simulink model "myGuyton_corrected_new"  (Simulink 6.6)
settings: Solver=ode15s  StartTime=0  StopTime=60*24*14  FixedStep=0.025  MaxStep=1  MinStep=0.00000001  RelTol=1e-1
values from neighbouring files (symbols this model uses):
  A1K = 0.5    [G92_var_decl_exp.m]
  A2K = 60    [G92_var_decl_exp.m]
  A3K = 40000    [G92_var_decl_exp.m]
  A4K = 0.1    [G92_var_decl_exp.m]
  A4K2 = 40000    [G92_var_decl_exp.m]
  AARK = 1    [G92_var_decl_exp.m]
  AARLL = 4    [G92_var_decl_exp.m]
  ADHC_IC = 1.01449    [G92_var_decl_exp.m]
  ADHINF = 0    [G92_var_decl_exp.m]
  ADHKLL = 0.2    [G92_var_decl_exp.m]
  ADHKUL = 5    [G92_var_decl_exp.m]
  ADHPAM = 0.3    [G92_var_decl_exp.m]
  ADHPUL = 85    [G92_var_decl_exp.m]
  ADHTC = 15    [G92_var_decl_exp.m]
  ADHVLL = 0.93617    [G92_var_decl_exp.m]
  ADHVUL = 2.5    [G92_var_decl_exp.m]
  AH10 = 0.333    [G92_var_decl_exp.m]
  AH11 = 1000    [G92_var_decl_exp.m]
  AH9 = 1    [G92_var_decl_exp.m]
  AHMNAR = 0.3    [G92_var_decl_exp.m]
  AHTHM = 2    [G92_var_decl_exp.m]
  AHY_IC = -0.461862    [G92_var_decl_exp.m]
  ALCLK = 0.3    [G92_var_decl_exp.m]
  ALDINF = 0    [G92_var_decl_exp.m]
  ALDKNS = 0    [G92_var_decl_exp.m]
  ALDMM = 2.5    [G92_var_decl_exp.m]
  AM1LL = 0    [G92_var_decl_exp.m]
  AM1UL = 5    [G92_var_decl_exp.m]
  AMC_IC = 1.05537    [G92_var_decl_exp.m]
  AMCSNS = 0.65    [G92_var_decl_exp.m]
  AMKM = 0.5    [G92_var_decl_exp.m]
  AMKMUL = 12    [G92_var_decl_exp.m]
  AMM1_IC = 1.00227    [G92_var_decl_exp.m]
  AMM2_IC = 1.09458    [G92_var_decl_exp.m]
  AMM4 = 0.005    [G92_var_decl_exp.m]
  AMNALL = 0.04    [G92_var_decl_exp.m]
  AMNAM = 0.8    [G92_var_decl_exp.m]
  AMNAUL = 15    [G92_var_decl_exp.m]
  AMT = 60    [G92_var_decl_exp.m]
  ANC_IC = 0.867681    [G92_var_decl_exp.m]
  ANCSNS = 0.4    [G92_var_decl_exp.m]
  ANGINF = 0    [G92_var_decl_exp.m]
  ANGKNS = 0    [G92_var_decl_exp.m]
  ANMALD = 2.5    [G92_var_decl_exp.m]
  ANMAM = 1.4    [G92_var_decl_exp.m]
  ANMARL = 0.86    [G92_var_decl_exp.m]
  ANMEM = 1.6    [G92_var_decl_exp.m]
  ANMKEL = 0.3    [G92_var_decl_exp.m]
  ANMKEM = 2    [G92_var_decl_exp.m]
  ANMLL = 0.7    [G92_var_decl_exp.m]
  ANMNAM = 1    [G92_var_decl_exp.m]
  ANMSLT = 2    [G92_var_decl_exp.m]
  ANMTM = 1.5    [G92_var_decl_exp.m]
  ANMUL = 1.8    [G92_var_decl_exp.m]
  ANPC_IC = 0.9333    [G92_var_decl_exp.m]
  ANPINF = 0    [G92_var_decl_exp.m]
  ANPKNS = 0    [G92_var_decl_exp.m]
  ANPTC = 4    [G92_var_decl_exp.m]
  ANPXAF = 1.5    [G92_var_decl_exp.m]
  ANPXUL = 10    [G92_var_decl_exp.m]
  ANT = 12    [G92_var_decl_exp.m]
  ANULL = 0.8    [G92_var_decl_exp.m]
  ANUM = 6    [G92_var_decl_exp.m]
  ANUVM = 0    [G92_var_decl_exp.m]
  ANV = 5000    [G92_var_decl_exp.m]
  ANX1_IC = 0    [G92_var_decl_exp.m]
  ANXM = 0    [G92_var_decl_exp.m]
  ANY = -0.2    [G92_var_decl_exp.m]
  AR1_IC = 1.00197    [G92_var_decl_exp.m]
  AR2_IC = 1.00306    [G92_var_decl_exp.m]
  AR3_IC = 1.05777    [G92_var_decl_exp.m]
  ARF = 0.5    [G92_var_decl_exp.m]
  ATRFBM = 0    [G92_var_decl_exp.m]
  ATRVM = 0    [G92_var_decl_exp.m]
  AU1_IC = 0.99999    [G92_var_decl_exp.m]
  AU4_IC = -0.00833091    [G92_var_decl_exp.m]
  AU6_IC = 1.00041    [G92_var_decl_exp.m]
  AUC1 = 0.3    [G92_var_decl_exp.m]
  AUDMP = 0.3    [G92_var_decl_exp.m]
  AUK = 0.004    [G92_var_decl_exp.m]
  AUL = 1.5    [G92_var_decl_exp.m]
  AULPM = 0    [G92_var_decl_exp.m]
  AUM1 = 3    [G92_var_decl_exp.m]
  AUM2 = 1    [G92_var_decl_exp.m]
  AUMAX = 5    [G92_var_decl_exp.m]
  AUMIN = 0.4    [G92_var_decl_exp.m]
  AUMK1 = 0.3    [G92_var_decl_exp.m]
  AUN1 = 0.5    [G92_var_decl_exp.m]
  AUS = 1    [G92_var_decl_exp.m]
  AUSLP = 1.5    [G92_var_decl_exp.m]
  AUTOGN = 7    [G92_var_decl_exp.m]
  AUTOK = 0.1    [G92_var_decl_exp.m]
  AUTOSN = 0.9    [G92_var_decl_exp.m]
  AUV = 0.55    [G92_var_decl_exp.m]
  AUX = 1    [G92_var_decl_exp.m]
  AUY = 0    [G92_var_decl_exp.m]
  BAROTC = 0.16    [G92_var_decl_exp.m]
  CFC = 0.01167    [G92_var_decl_exp.m]
  CKEEX = 4    [G92_var_decl_exp.m]
  CMPTSS = 2    [G92_var_decl_exp.m]
  CN2 = 0.0212    [G92_var_decl_exp.m]
  CN3_IC = 0.359907    [G92_var_decl_exp.m]
  CN7 = 0.2    [G92_var_decl_exp.m]
  CNR = 139    [G92_var_decl_exp.m]
  CPF = 0.0003    [G92_var_decl_exp.m]
  CPK = 0.000253    [G92_var_decl_exp.m]
  CPR = 40    [G92_var_decl_exp.m]
  CRRFLX = 0    [G92_var_decl_exp.m]
  CV = 0.1    [G92_var_decl_exp.m]
  DFP_IC = 1.16492e-06    [G92_var_decl_exp.m]
  DHDTR = 0.05    [G92_var_decl_exp.m]
  DIURET = 1    [G92_var_decl_exp.m]
  DR = 0    [G92_var_decl_exp.m]
  DTKA_IC = 0.0368507    [G92_var_decl_exp.m]
  DTNAR = 0.675    [G92_var_decl_exp.m]
  DTNARL = 1e-06    [G92_var_decl_exp.m]
  EARK = 1    [G92_var_decl_exp.m]
  EARLL = 24    [G92_var_decl_exp.m]
  EFAFR = 0    [G92_var_decl_exp.m]
  EXC = 1    [G92_var_decl_exp.m]
  ... (+137 more)
libraries: simulink x5
(part 1 of 3)
settings Model: Creator=Villy  LastModifiedBy=Villy
settings DataIOCC: LimitDataPoints=off  SaveOutput=off  SaveTime=off
settings DebuggingCC: SignalInfNanChecking=error  AlgebraicLoopMsg=none  ArtificialAlgebraicLoopMsg=error  SignalResolutionControl=TryResolveAll  BlockPriorityViolationMsg=error  MinStepSizeMsg=error  SolverPrmCheckMsg=error

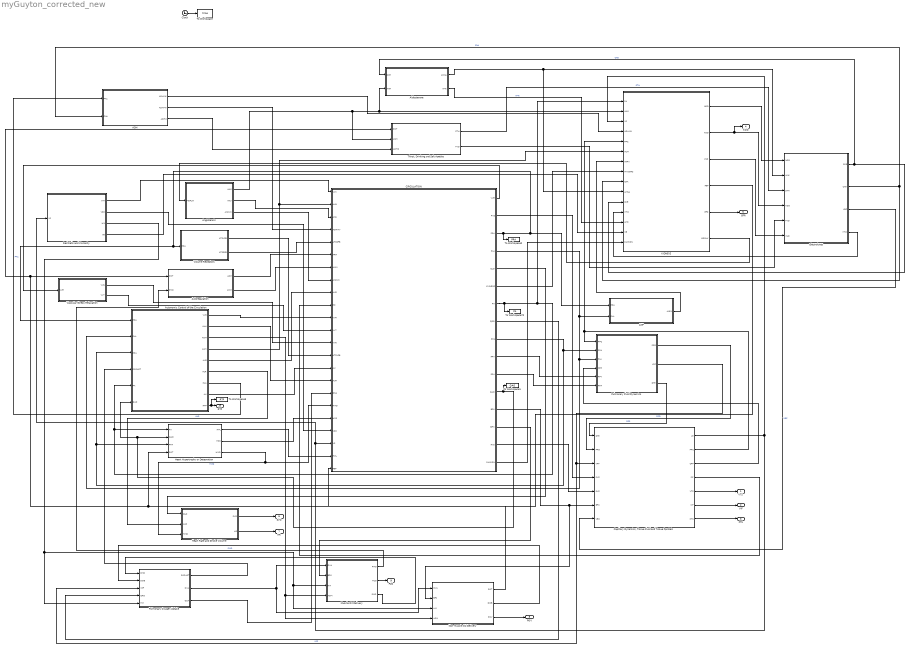
== system myGuyton_corrected_new ==
  ADH : Subsystem
      mask Display: disp('ANTIDIURETIC HORMONE')
  ANP : Subsystem
      mask Display: disp('ATRIAL NATRIURETIC PEPTIDE')
  Aldosterone : Subsystem
      mask Display: disp('ALDOSTERONE')
  Angiotensin : Subsystem
      mask Display: disp('ANGIOTENSIN')
  Autonomic Control of the Circulation : Subsystem
      mask Display: disp('AUTONOMICS')
  Autoregulation : Subsystem
      mask Display: disp('Autoregulatory Local Blood Flow Control')
  CIRCULATION : Subsystem
      mask Display: disp('CIRCULATORY DYNAMICS')
  "Capillary Dynamics, Tissue Fluid and Tissue Pprotein " : Subsystem
      mask Display: disp('CAPILLARY DYNAMICS, TISSUE FLUID AND TISSUE PROTEIN')
  Clock : Clock
      settings: Decimation=10
  Electrolytes : Subsystem
      mask Display: disp('ELECTROLYTES')
  Heart Hypertrophy or Deteoration : Subsystem
      mask Display: disp('Heart Hypertrophy or Deteoration')
  Heart Rate and Stroke Volume : Subsystem
      mask Display: disp('Heart Rate and Stroke Volume')
  KIDNEYS : Subsystem
      mask Display: disp('KIDNEYS')
  Muscle O2 Delivery : Subsystem
      mask Display: disp('MUSCLE OXYGEN DELIVERY')
  Non-muscle O2 Delivery : Subsystem
      mask Display: disp('NON-MUSCLE OXYGEN DELIVERY')
  Pulmonary Fluid Dynamics : Subsystem
      mask Display: disp('PULMONARY FLUID DYNAMICS')
  Pulmonary Oxygen Uptake : Subsystem
      mask Display: disp('PULMONARY 02 UPTAKE')
  Red Cells and Viscosity : Subsystem
      mask Display: disp('RED CELLS AND VISCOSITY')
  "Thirst, Drinking snd Salt Apetite" : Subsystem
      mask Display: disp('THURST, DRINKING AND SALT APETITE')
  To Workspace : ToWorkspace  VariableName=time  SampleTime=-1  SaveFormat=Array
  To Workspace1 : ToWorkspace  VariableName=QAO  SampleTime=-1  SaveFormat=Array
  To Workspace2 : ToWorkspace  VariableName=PRA  SampleTime=-1  SaveFormat=Array
  To Workspace3 : ToWorkspace  VariableName=RTP  SampleTime=-1  SaveFormat=Array
  To Workspace72 : ToWorkspace  VariableName=PA  SampleTime=-1  SaveFormat=Array
  Vascular Stress Relaxation : Subsystem
      mask Display: disp('Stress Relaxation')
  Volume Receptors : Subsystem
      mask Display: disp('Volume Receptors')
  VTS : Outport
  VIF : Outport  Port=2
  PTS : Outport  Port=3
  KOD : Outport  Port=4
  GFR : Outport  Port=5
  SVO : Outport  Port=6
  HR : Outport  Port=7
  POV : Outport  Port=8
  P2O : Outport  Port=9
  RTP : Outport  Port=10
  wires:
  CIRCULATION/4(PLA) -> Autonomic Control of the Circulation/2(PLA), Pulmonary Fluid Dynamics/3(PLA), ANP/2(PLA)
  CIRCULATION/2(PVS) -> "Capillary Dynamics, Tissue Fluid and Tissue Pprotein "/4(PVS)
  CIRCULATION/3(PRA) -> ANP/1(PRA), Volume Receptors/1(PRA), Autonomic Control of the Circulation/1(PRA), To Workspace2/1
  CIRCULATION/5(QLO) -> Heart Rate and Stroke Volume/1(QLO)
  CIRCULATION/6(MYOGRS) -> KIDNEYS/8(MYOGRS)
  CIRCULATION/7(PA) -> KIDNEYS/1(PA), Autonomic Control of the Circulation/5(PA), Heart Hypertrophy or Deteoration/1(PA), To Workspace72/1
  CIRCULATION/8(QRO) -> Pulmonary Oxygen Uptake/4(QRO)
  CIRCULATION/9(PPA) -> Pulmonary Fluid Dynamics/2(PPA), Autonomic Control of the Circulation/3(PPA), Heart Hypertrophy or Deteoration/3(PPA)
  CIRCULATION/10(RPV) -> Pulmonary Fluid Dynamics/5(RPV)
  CIRCULATION/11(RPA) -> Pulmonary Fluid Dynamics/6(RPA)
  CIRCULATION/13(BFN) -> "Capillary Dynamics, Tissue Fluid and Tissue Pprotein "/6(BFN), Non-muscle O2 Delivery/2(BFN)
  CIRCULATION/14(BFM) -> Muscle O2 Delivery/2(BFM)
  Autonomic Control of the Circulation/2(AUH) -> CIRCULATION/16(AUH)
  Autonomic Control of the Circulation/6(AUR) -> Heart Rate and Stroke Volume/2(AUR)  "AUR"
  Autonomic Control of the Circulation/3(AOM) -> Muscle O2 Delivery/4(AOM), Non-muscle O2 Delivery/4(AOM)
  Autonomic Control of the Circulation/4(AUM) -> CIRCULATION/2(AUM), KIDNEYS/6(AUM)
  Autonomic Control of the Circulation/5(AVE) -> CIRCULATION/9(AVE)
  Autonomic Control of the Circulation/1(VVR) -> CIRCULATION/11(VVR)
  Autonomic Control of the Circulation/7(PA1) -> ADH/1(PA1)  "PA1"
  Autonomic Control of the Circulation/8(AU) -> CIRCULATION/15(AU)
  Angiotensin/3(ANUVN) -> CIRCULATION/8(ANUVN)
  Angiotensin/1(ANM) -> KIDNEYS/2(ANM), Aldosterone/2(ANM), "Thirst, Drinking snd Salt Apetite"/2(ANM)
  Angiotensin/2(ANU) -> CIRCULATION/3(ANU)
  Volume Receptors/2(ATRRFB) -> CIRCULATION/5(ATRRFB)
  Volume Receptors/1(ATRVFB) -> CIRCULATION/14(ATRVFB)
  Autoregulation/2(AMM) -> CIRCULATION/7(AMM)
  Autoregulation/1(ARM) -> CIRCULATION/6(ARM)
  Vascular Stress Relaxation/1(VV6) -> CIRCULATION/13(VV6)
  Vascular Stress Relaxation/2(VV7) -> CIRCULATION/12(VV7)
  Pulmonary Fluid Dynamics/1(PPD) -> "Capillary Dynamics, Tissue Fluid and Tissue Pprotein "/2(PPD)  "PPD"
  Pulmonary Fluid Dynamics/2(VPF) -> "Capillary Dynamics, Tissue Fluid and Tissue Pprotein "/3(VPF), Pulmonary Oxygen Uptake/3(VPF)  "VPF"
  Pulmonary Fluid Dynamics/3(DFP) -> "Capillary Dynamics, Tissue Fluid and Tissue Pprotein "/1(DFP)  "DFP"
  "Capillary Dynamics, Tissue Fluid and Tissue Pprotein "/2(PPC) -> Pulmonary Fluid Dynamics/1(PPC), KIDNEYS/5(PPC)
  "Capillary Dynamics, Tissue Fluid and Tissue Pprotein "/3(CPP) -> Pulmonary Fluid Dynamics/4(CPP)
  "Capillary Dynamics, Tissue Fluid and Tissue Pprotein "/5(VTS) -> VTS/1
  "Capillary Dynamics, Tissue Fluid and Tissue Pprotein "/4(PC) -> CIRCULATION/10(PC)
  "Capillary Dynamics, Tissue Fluid and Tissue Pprotein "/6(VIF) -> VIF/1
  "Capillary Dynamics, Tissue Fluid and Tissue Pprotein "/7(PTS) -> PTS/1
  "Capillary Dynamics, Tissue Fluid and Tissue Pprotein "/1(VP) -> KIDNEYS/3(VP), CIRCULATION/21(VP), Red Cells and Viscosity/1(VP)
  CIRCULATION/15(RVS) -> "Capillary Dynamics, Tissue Fluid and Tissue Pprotein "/5(RVS)
  KIDNEYS/1(NOD) -> Electrolytes/1(NOD)
  KIDNEYS/2(KOD) -> KOD/1, Electrolytes/4(KOD)
  KIDNEYS/3(VUD) -> Electrolytes/6(VUD)
  KIDNEYS/4(RBF) -> CIRCULATION/23(RBF)
  KIDNEYS/5(GFR) -> GFR/1
  KIDNEYS/6(MDFLW) -> Angiotensin/1(MDFLW)
  Electrolytes/1(CKE) -> KIDNEYS/11(CKE), Aldosterone/1(CKE)  "CKE"
  Electrolytes/2(CNA) -> KIDNEYS/9(CNA), ADH/2(CNA)  "CNA"
  Electrolytes/3(VEC) -> "Capillary Dynamics, Tissue Fluid and Tissue Pprotein "/7(VEC)  "VEC"
  Electrolytes/4(VTW) -> KIDNEYS/12(VTW)
  ADH/1(ADHMK) -> KIDNEYS/4(ADHMK)
  ADH/2(ADHMV) -> CIRCULATION/4(ADHMV)
  ADH/3(ADHC) -> "Thirst, Drinking snd Salt Apetite"/3(ADHC)
  Aldosterone/2(AMK) -> KIDNEYS/13(AMK)  "AMK"
  Aldosterone/1(AMNA) -> KIDNEYS/10(AMNA), Electrolytes/2(AMK)
  ANP/1(ANPX) -> KIDNEYS/7(ANPX)
  Heart Rate and Stroke Volume/1(SVO) -> SVO/1
  Heart Rate and Stroke Volume/2(HR) -> HR/1
  "Thirst, Drinking snd Salt Apetite"/2(TVD) -> Electrolytes/5(TVD)
  "Thirst, Drinking snd Salt Apetite"/1(STH) -> Electrolytes/3(STH)  "STH"
  Red Cells and Viscosity/1(VIM) -> CIRCULATION/1(VIM)
  Red Cells and Viscosity/2(VRC) -> CIRCULATION/20(VRC)
  Red Cells and Viscosity/3(HM) -> Muscle O2 Delivery/3(HM), Non-muscle O2 Delivery/3(HM), Pulmonary Oxygen Uptake/5(HM)
  Red Cells and Viscosity/4(VB) -> KIDNEYS/14(VB)
  Muscle O2 Delivery/1(PMO) -> Autoregulation/2(PMO)  "PMO"
  Muscle O2 Delivery/2(P2O) -> P2O/1
  Muscle O2 Delivery/3(RMO) -> Pulmonary Oxygen Uptake/1(RMO)
  Non-muscle O2 Delivery/1(POT) -> Heart Hypertrophy or Deteoration/4(POT), Autoregulation/1(POT), "Thirst, Drinking snd Salt Apetite"/1(POT)
  Non-muscle O2 Delivery/2(DOB) -> Pulmonary Oxygen Uptake/2(DOB)
  Non-muscle O2 Delivery/3(POV) -> POV/1
  Pulmonary Oxygen Uptake/1(PO2ART) -> Autonomic Control of the Circulation/4(PO2ART)
  Pulmonary Oxygen Uptake/2(OVA) -> Muscle O2 Delivery/1(OVA), Non-muscle O2 Delivery/1(OVA)
  Pulmonary Oxygen Uptake/3(OSA) -> CIRCULATION/17(OSA)
  CIRCULATION/16(PAMKRN) -> KIDNEYS/15(PAMKRN)
  Heart Hypertrophy or Deteoration/3(HMD) -> CIRCULATION/18(HMD), Heart Rate and Stroke Volume/3(HMD)  "HMD"
  Heart Hypertrophy or Deteoration/1(HPL) -> CIRCULATION/22(HPL)
  Heart Hypertrophy or Deteoration/2(HPR) -> CIRCULATION/19(HPR)
  CIRCULATION/1(VVE) -> Vascular Stress Relaxation/1(VVE)
  CIRCULATION/12(QAO) -> To Workspace1/1, Heart Hypertrophy or Deteoration/2(QAO), Autonomic Control of the Circulation/6(QAO)
  Clock/1 -> To Workspace/1
  Autonomic Control of the Circulation/9(RTP) -> RTP/1, To Workspace3/1

== system myGuyton_corrected_new/ADH ==
  note: ADHC = ADH CONCENTRATION
      | (RATIO TO NORMAL)
  PA1 : Inport
  CNA : Inport  Port=2
  ADH (TOTAL ADH SECRETION) : Subsystem
      mask Display: disp('ADH CALCULATION')
  ADH Concentration : Subsystem
      mask Display: dpoly([0 1],[ADHTC*Z16 1])
  ADHMK = ADH EFFECT ON SODIUM AND  WATER REABSORPTION : Subsystem
      mask Display: disp('ADHMK CALCULATION')
  ADHMV = ADH EFFECT ON NONRENAL  VASCULAR RESISTANCE : Subsystem
      mask Display: disp('ADHMV CALCULATION')
  ADHMK : Outport
  ADHMV : Outport  Port=2
  ADHC : Outport  Port=3
  wires:
  ADH (TOTAL ADH SECRETION)/1(ADH) -> ADH Concentration/1(ADH)  "ADH"
  ADH Concentration/1(ADHC) -> ADHMK = ADH EFFECT ON SODIUM AND  WATER REABSORPTION/1(ADHC), ADHMV = ADH EFFECT ON NONRENAL  VASCULAR RESISTANCE/1(ADHC), ADHC/1  "ADHC"
  PA1/1 -> ADH (TOTAL ADH SECRETION)/1(PA1)
  ADHMK = ADH EFFECT ON SODIUM AND  WATER REABSORPTION/1(ADHMK) -> ADHMK/1
  CNA/1 -> ADH (TOTAL ADH SECRETION)/2(CNA)
  ADHMV = ADH EFFECT ON NONRENAL  VASCULAR RESISTANCE/1(ADHMV) -> ADHMV/1

== system myGuyton_corrected_new/ANP ==
  PRA : Inport
  PLA : Inport  Port=2
  ANP ACCUMULATION  AND DESTRUCTION : Subsystem
      mask Display: dpoly([0 1], [ANPTC*Z14 1])
  Constant : Constant
  Constant1 : Constant  Value=ANPINF
  Constant2 : Constant  Value=ANPKNS
  Constant3 : Constant  Value=ANPXUL
  Constant4 : Constant
  Divide : Product  Inputs=*/  OutScaling=2^-10
  Gain : Gain  Gain=2
  Gain1 : Gain  Gain=1/3
  Gain2 : Gain  Gain=0.5555556
  "IF ANPKNS>0, ANP1=ANPKNS ELSE, ANP1 = ANP1 " : Switch  Criteria=u2 > Threshold
  Saturation : Saturate  UpperLimit=inf  LowerLimit=0
  Saturation1 : Saturate  UpperLimit=inf  LowerLimit=0
  Saturation2 : Saturate  UpperLimit=inf  LowerLimit=-1
  Sum : Sum  Inputs=|++
  Sum1 : Sum  Inputs=-+|
  Sum2 : Sum
  Sum3 : Sum  Inputs=++|
  Sum4 : Sum  Inputs=|+-
  Sum5 : Sum  Inputs=|++
  ANPX : Outport
  wires:
  Constant/1 -> Sum/2, Sum1/1
  Sum1/1 -> Saturation/1  "ANPL"
  Sum/1 -> Gain/1
  Gain/1 -> Saturation1/1  "ANPR2"
  Saturation1/1 -> Sum2/1
  Saturation/1 -> Sum2/2  "ANPL"
  Sum2/1 -> Gain1/1
  Gain1/1 -> Sum3/2  "ANP"
  Constant1/1 -> Sum3/1
  Sum3/1 -> "IF ANPKNS>0, ANP1=ANPKNS ELSE, ANP1 = ANP1 "/3  "ANP1"
  Constant2/1 -> "IF ANPKNS>0, ANP1=ANPKNS ELSE, ANP1 = ANP1 "/2, "IF ANPKNS>0, ANP1=ANPKNS ELSE, ANP1 = ANP1 "/1
  "IF ANPKNS>0, ANP1=ANPKNS ELSE, ANP1 = ANP1 "/1 -> ANP ACCUMULATION  AND DESTRUCTION/1(ANP1)  "ANP1"
  ANP ACCUMULATION  AND DESTRUCTION/1(ANPC) -> Sum5/1  "ANPC"
  Constant3/1 -> Sum4/1, Divide/1  "ANPXUL"
  Constant4/1 -> Sum5/2
  Sum5/1 -> Gain2/1
  Gain2/1 -> Divide/2
  Divide/1 -> Sum4/2
  Sum4/1 -> Saturation2/1
  PRA/1 -> Sum/1
  PLA/1 -> Sum1/2
  Saturation2/1 -> ANPX/1  "ANPX"

== system myGuyton_corrected_new/Aldosterone ==
  note: AM
  note: AMK
  CKE : Inport
  ANM : Inport  Port=2
  AM1 : Subsystem
      mask Display: disp('AM1 CALCULATION')
  AMR1 : Subsystem
      mask Display: disp('AMR1 CALCULATION')
  AMRBSC : Subsystem
      mask Display: disp('AMRBSC CALCULATION')
  Aldost. Concentration Dynamics : Subsystem
      mask Display: dpoly([0 1], [AMT 1])
  Constant : Constant
  Constant1 : Constant
  Gain : Gain  Gain=ALDMM
  Gain1 : Gain  Gain=AMKM
  Gain2 : Gain  Gain=AMNAM
  Saturation : Saturate  UpperLimit=inf  LowerLimit=0.2
  Saturation1 : Saturate  UpperLimit=AMNAUL  LowerLimit=AMNALL
  Sum1 : Sum  Inputs=|++
  Sum12 : Sum  Inputs=|+-
  Sum2 : Sum  Inputs=|+-
  Sum3 : Sum  Inputs=|++
  Sum4 : Sum  Inputs=|++
  AMNA : Outport
  AMK : Outport  Port=2
  wires:
  AMRBSC/1(AMRBSC) -> AMR1/1(AMRBSC)  "AMRBSC"
  AMR1/1(AMR1) -> Aldost. Concentration Dynamics/1(AMR1)  "AMR1"
  Aldost. Concentration Dynamics/1(AMC) -> AM1/1(AMC)  "AMC"
  AM1/1(AM1) -> Sum12/1  "AM1"
  Constant/1 -> Sum12/2, Sum1/2, Sum2/2, Sum3/2
  Sum12/1 -> Gain/1
  Gain/1 -> Sum1/1
  Sum1/1 -> Sum2/1
  Sum2/1 -> Gain1/1, Gain2/1  "AM-1"
  Gain1/1 -> Sum3/1
  Sum3/1 -> Saturation/1
  Constant1/1 -> Sum4/2
  Gain2/1 -> Sum4/1
  Sum4/1 -> Saturation1/1
  ANM/1 -> AMRBSC/2(ANM)
  Saturation1/1 -> AMNA/1  "AMNA"
  CKE/1 -> AMRBSC/1(CKE)
  Saturation/1 -> AMK/1

== system myGuyton_corrected_new/Angiotensin ==
  note: ANPR1
  note: ANU
  MDFLW : Inport
  0.00001 : Saturate  UpperLimit=inf  LowerLimit=0.00001
  ANG Secretion Dynamics : Subsystem
      mask Display: dpoly([0 1], [ANV 1])
  ANM Calculation : Subsystem
      mask Display: disp('ANM CALCULATION')
  ANULL : Saturate  UpperLimit=inf  LowerLimit=ANULL
  Angiotensin Secretion  Due to MD Flow : Subsystem
      mask Display: disp('ANGSCR CALCULATION')
  Constant : Constant  Value=ANGINF
  Constant1 : Constant  Value=ANGKNS
  Constant2 : Constant  Orientation=up
  Constant6 : Constant  Orientation=up
  Gain1 : Gain  Gain=REK
  Gain2 : Gain  Gain=ANUM
  Gain3 : Gain  Gain=ANXM
  Gain4 : Gain  Gain=ANUVM
  "IF ANGKNS>0, ANPR1=ANGKNS ELSE ANPR1 = ANPR1" : Switch  Criteria=u2 > Threshold
  MDFLW3 : Subsystem
      mask Display: dpoly([0 1],[MDFLWX 1])
  Plasma ANG Concentration : Subsystem
      mask Display: dpoly([0 1],[ANT 1])
  Sum{1,3..4,7} (4 alike) : Sum  Inputs=|++
  Sum2 : Sum  Inputs=|+-
  Sum5 : Sum  Inputs=|+-
  Sum6 : Sum  Inputs=|+-
  ANM : Outport
  ANU : Outport  Port=2
  ANUVN : Outport  Port=3
  wires:
  MDFLW3/1(MDFLW3) -> Angiotensin Secretion  Due to MD Flow/1(MDFLW3)  "MDFLW3"
  ANG Secretion Dynamics/1(ANX1) -> Sum1/1  "ANX1"
  Constant6/1 -> Sum6/2
  Sum6/1 -> Gain3/1
  Gain3/1 -> ANG Secretion Dynamics/1(ANX)  "ANX"
  Angiotensin Secretion  Due to MD Flow/1(ANGSCR) -> Sum6/1, Sum1/2  "ANGSCR"
  Sum1/1 -> Gain1/1
  Gain1/1 -> 0.00001/1  "ANPR"
  0.00001/1 -> Sum3/1
  Constant/1 -> Sum3/2
  Sum3/1 -> "IF ANGKNS>0, ANPR1=ANGKNS ELSE ANPR1 = ANPR1"/3
  Constant1/1 -> "IF ANGKNS>0, ANPR1=ANGKNS ELSE ANPR1 = ANPR1"/2, "IF ANGKNS>0, ANPR1=ANGKNS ELSE ANPR1 = ANPR1"/1
  "IF ANGKNS>0, ANPR1=ANGKNS ELSE ANPR1 = ANPR1"/1 -> Plasma ANG Concentration/1(ANPR1)  "ANPR1"
  Plasma ANG Concentration/1(ANC) -> ANM Calculation/1(ANC)  "ANC"
  ANM Calculation/1(ANM) -> Sum2/1, ANM/1  "ANM"
  Constant2/1 -> Sum2/2, Sum4/2, Sum5/2, Sum7/2
  Sum2/1 -> Gain2/1  "ANM-1"
  Gain2/1 -> Sum4/1
  Sum4/1 -> ANULL/1  "ANU"
  ANULL/1 -> Sum5/1, ANU/1  "ANU"
  Sum5/1 -> Gain4/1
  Gain4/1 -> Sum7/1
  MDFLW/1 -> MDFLW3/1(MDFLW)
  Sum7/1 -> ANUVN/1  "ANUVN"

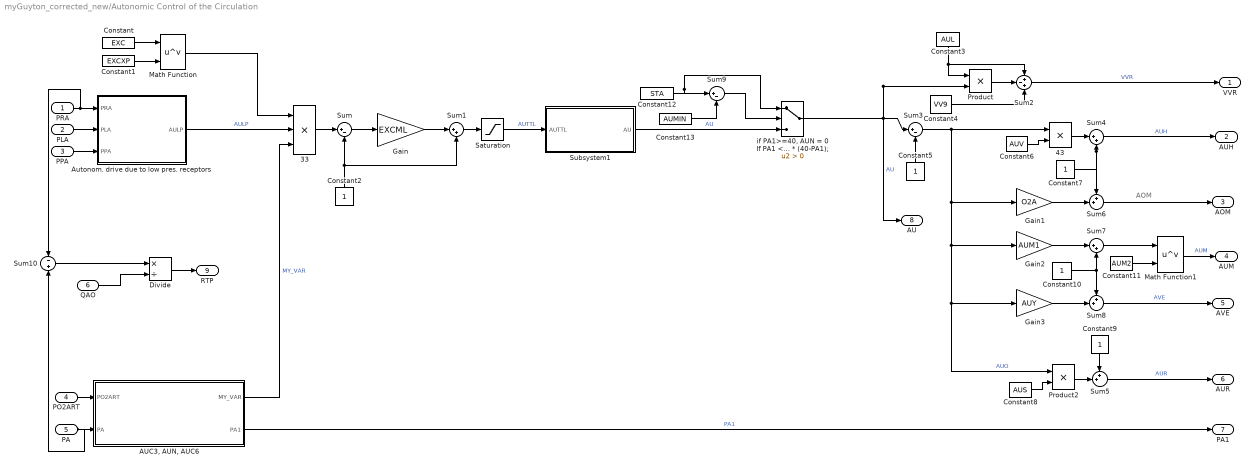
== system myGuyton_corrected_new/Autonomic Control of the Circulation ==
  note: AOM
  PRA : Inport
  PLA : Inport  Port=2
  PPA : Inport  Port=3
  PO2ART : Inport  Port=4
  PA : Inport  Port=5
  QAO : Inport  Port=6
  33 : Product  Inputs=3  RndMeth=Zero
  43 : Product  RndMeth=Zero
  "AUC3, AUN, AUC6" : Subsystem
      mask Display: disp('CALCULATION OF AUC3, AUN AND AUC6')
  "Autonom. drive due to low pres. receptors " : Subsystem
      mask Display: disp('AULP CALCULATION')
  Constant : Constant  Value=EXC
  Constant1 : Constant  Value=EXCXP
  Constant10 : Constant
  Constant11 : Constant  Value=AUM2
  Constant12 : Constant  Value=STA
  Constant13 : Constant  Value=AUMIN
  Constant2 : Constant  Orientation=up
  Constant3 : Constant  Orientation=down  Value=AUL
  Constant4 : Constant  Value=VV9
  Constant5 : Constant  Orientation=up
  Constant6 : Constant  Value=AUV
  Constant7 : Constant
  Constant8 : Constant  Value=AUS
  Constant9 : Constant  Orientation=down
  Divide : Product  Inputs=*/  OutScaling=2^-10
  Gain : Gain  Gain=EXCML
  Gain1 : Gain  Gain=O2A
  Gain2 : Gain  Gain=AUM1
  Gain3 : Gain  Gain=AUY
  Math Function : Math  Operator=pow  SaturateOnIntegerOverflow=on
  Math Function1 : Math  Operator=pow  SaturateOnIntegerOverflow=on
  Product : Product  RndMeth=Zero
  Product2 : Product  RndMeth=Zero
  Saturation : Saturate  UpperLimit=inf  LowerLimit=0  LinearizeAsGain=off
  Subsystem1 : Subsystem
      mask Display: disp('AU CALCULATION')
  Sum : Sum  Inputs=|+-
  Sum1 : Sum  Inputs=|++
  Sum10 : Sum  Inputs=-+
  Sum2 : Sum  Inputs=+-+
  Sum3 : Sum  Inputs=|+-
  Sum4 : Sum  Inputs=|++
  Sum5 : Sum  Inputs=++|
  Sum6 : Sum  Inputs=++|
  Sum7 : Sum  Inputs=|++
  Sum8 : Sum  Inputs=++|
  Sum9 : Sum  Inputs=|+-
  "if PA1>=40, AUN = 0 If PA1 < 40, AUN = 0.04 * (40-PA1);" : Switch  Criteria=u2 > Threshold
  VVR : Outport
  AUH : Outport  Port=2
  AOM : Outport  Port=3
  AUM : Outport  Port=4
  AVE : Outport  Port=5
  AUR : Outport  Port=6
  PA1 : Outport  Port=7
  AU : Outport  Port=8
  RTP : Outport  Port=9
  wires:
  "AUC3, AUN, AUC6"/1(MY_VAR) -> 33/3  "MY_VAR"
  "Autonom. drive due to low pres. receptors "/1(AULP) -> 33/2  "AULP"
  Constant/1 -> Math Function/1
  Constant1/1 -> Math Function/2
  Math Function/1 -> 33/1
  Constant2/1 -> Sum/2, Sum1/2
  33/1 -> Sum/1
  Sum/1 -> Gain/1
  Gain/1 -> Sum1/1
  Saturation/1 -> Subsystem1/1(AUTTL)  "AUTTL"
  Sum1/1 -> Saturation/1
  Subsystem1/1(AU) -> "if PA1>=40, AUN = 0 If PA1 < 40, AUN = 0.04 * (40-PA1);"/3  "AU"
  Constant3/1 -> Product/1, Sum2/1
  Product/1 -> Sum2/2
  Sum2/1 -> VVR/1  "VVR"
  Constant4/1 -> Sum2/3
  Constant5/1 -> Sum3/2
  Sum3/1 -> 43/1, Gain1/1, Gain2/1, Product2/1, Gain3/1  "AUO"
  Constant6/1 -> 43/2
  43/1 -> Sum4/1
  Constant7/1 -> Sum4/2, Sum6/1
  Constant8/1 -> Product2/2
  Product2/1 -> Sum5/2
  Constant9/1 -> Sum5/1
  Gain1/1 -> Sum6/2
  Gain2/1 -> Sum7/1
  Constant10/1 -> Sum7/2, Sum8/1
  Gain3/1 -> Sum8/2
  Sum7/1 -> Math Function1/1
  Constant11/1 -> Math Function1/2
  PRA/1 -> "Autonom. drive due to low pres. receptors "/1(PRA), Sum10/1
  PPA/1 -> "Autonom. drive due to low pres. receptors "/3(PPA)
  PA/1 -> "AUC3, AUN, AUC6"/2(PA), Sum10/2
  PLA/1 -> "Autonom. drive due to low pres. receptors "/2(PLA)
  Sum4/1 -> AUH/1  "AUH"
  Sum6/1 -> AOM/1
  PO2ART/1 -> "AUC3, AUN, AUC6"/1(PO2ART)
  Math Function1/1 -> AUM/1  "AUM"
  Sum8/1 -> AVE/1  "AVE"
  Sum5/1 -> AUR/1  "AUR"
  "AUC3, AUN, AUC6"/2(PA1) -> PA1/1  "PA1"
  Sum9/1 -> "if PA1>=40, AUN = 0 If PA1 < 40, AUN = 0.04 * (40-PA1);"/2
  Constant13/1 -> Sum9/2
  Constant12/1 -> Sum9/1, "if PA1>=40, AUN = 0 If PA1 < 40, AUN = 0.04 * (40-PA1);"/1
  "if PA1>=40, AUN = 0 If PA1 < 40, AUN = 0.04 * (40-PA1);"/1 -> Product/2, Sum3/1, AU/1  "AU"
  Sum10/1 -> Divide/1
  QAO/1 -> Divide/2
  Divide/1 -> RTP/1

== system myGuyton_corrected_new/Autoregulation ==
  POT : Inport
  PMO : Inport  Port=2
  Muscle Local BF Control : Subsystem
      mask Display: disp('Muscle Local BF Control')
  Non-Muscle Local BF Control : Subsystem
      mask Display: disp('Non-Muscle Local BF Control')
  ARM : Outport
  AMM : Outport  Port=2
  wires:
  POT/1 -> Non-Muscle Local BF Control/1(POT)
  Non-Muscle Local BF Control/1(ARM) -> ARM/1
  PMO/1 -> Muscle Local BF Control/1(PMO)
  Muscle Local BF Control/1(AMM) -> AMM/1

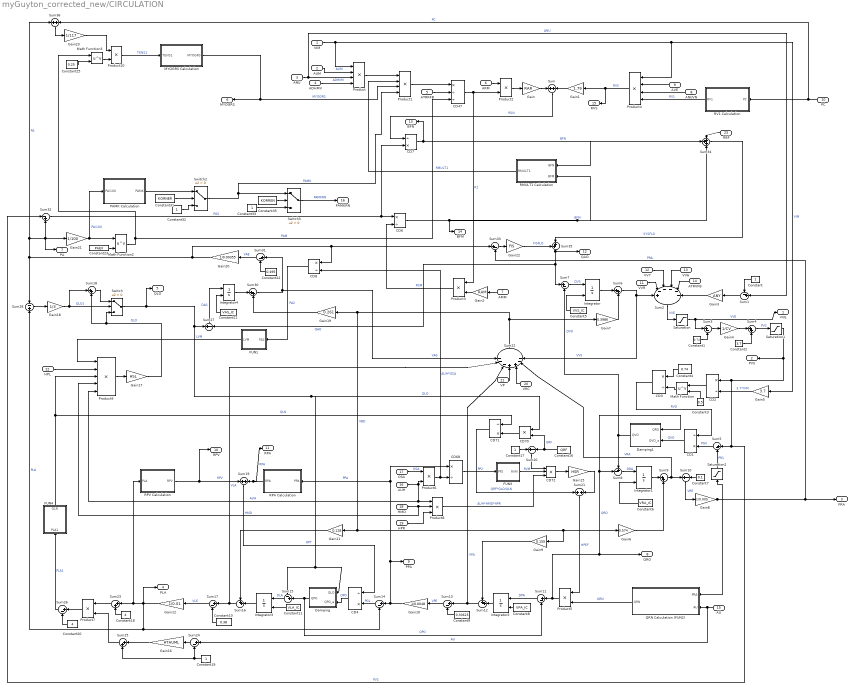
== system myGuyton_corrected_new/CIRCULATION ==
  VIM : Inport
  AUM : Inport  Port=2
  ANU : Inport  Port=3
  ADHMV : Inport  Port=4
  ATRRFB : Inport  Port=5
  ARM : Inport  Port=6
  AMM : Inport  Orientation=left  Port=7
  ANUVN : Inport  Orientation=left  Port=8
  AVE : Inport  Orientation=left  Port=9
  PC : Inport  Orientation=left  Port=10
  VVR : Inport  Port=11
  VV7 : Inport  Port=12
  VV6 : Inport  Orientation=left  Port=13
  ATRVFB : Inport  Orientation=left  Port=14
  AU : Inport  Orientation=left  Port=15
  AUH : Inport  Port=16
  OSA : Inport  Port=17
  HMD : Inport  Port=18
  HPR : Inport  Port=19
  VRC : Inport  Orientation=left  Port=20
  VP : Inport  Port=21
  HPL : Inport  Port=22
  RBF : Inport  Orientation=left  Port=23
  CD1 : Product  Orientation=left  Inputs=/*  OutScaling=2^-10
  CD2 : Product  Orientation=left  Inputs=*/  OutScaling=2^-10
  CD3 : Product  Orientation=left  Inputs=*/  OutScaling=2^-10
  CD4 : Product  Orientation=left  Inputs=/*  OutScaling=2^-10
  CD47 : Product  Inputs=*//  OutScaling=2^-10
  CD6 : Product  Inputs=*/  OutScaling=2^-10
  CD68 : Product  Inputs=*/  OutScaling=2^-10
  CD7 : Product  Inputs=/*  OutScaling=2^-10
  CD70 : Product  Orientation=left  RndMeth=Zero
  CD71 : Product  Orientation=left  Inputs=/*  OutScaling=2^-10
  CD72 : Product  Inputs=3  RndMeth=Zero
  CD8 : Product  Orientation=left  Inputs=*/  OutScaling=2^-10
  Constant : Constant  Orientation=left
  Constant1 : Constant  Value=0.74
  Constant10 : Constant  Orientation=left  Value=0.38
  Constant11 : Constant  Orientation=left  Value=VLA_IC
  Constant16 : Constant  Orientation=left  Value=QRF
  Constant17 : Constant
  Constant18 : Constant  Orientation=left  Value=4
  Constant19 : Constant  Orientation=left
  Constant2 : Constant  Value=3.7
  Constant20 : Constant  Orientation=left  Value=4
  Constant21 : Constant  Orientation=left  Value=VAS_IC
  Constant22 : Constant  Orientation=left  Value=0.495
  Constant23 : Constant  Value=PAEX
  Constant25 : Constant  Value=0.25
  Constant3 : Constant  Orientation=up  Value=0.5
  Constant31 : Constant  Value=KORNER
  Constant32 : Constant
  Constant33 : Constant
  Constant35 : Constant  Value=KORREN
  Constant4 : Constant  Orientation=left  Value=0.74
  Constant5 : Constant  Orientation=left  Value=VVS_IC
  Constant6 : Constant  Orientation=left  Value=VRA_IC
  Constant7 : Constant  Orientation=left  Value=0.1
  Constant8 : Constant  Orientation=left  Value=VPA_IC
  Constant9 : Constant  Orientation=left  Value=0.30625
  Damping : Subsystem  Orientation=left
  Damping1 : Subsystem  Orientation=left
  FUN1 : Subsystem  Orientation=left
      mask Display: plot([0,  60 , 125,  160, 200, 240 ], [1.04, 1.025, 0.97, 0.88, 0.59, 0] )
  FUN3 : Subsystem
      mask Display: plot([0,  32, 38.4, 48.0, 60.8, 72.0], [1.06,  0.97,   0.93,  0.8,  0.46,  0.0])
  FUN4 : Subsystem  Orientation=up
      mask Display: plot([-2, 1, 5, 8, 12], [0.01, 3.6, 9.4, 11.6, 13.5])
  Gain : Gain  Gain=RAR
  Gain1 : Gain  Orientation=left  Gain=1.79
  Gain10 : Gain  Orientation=left  Gain=1/0.0048
  Gain11 : Gain  Orientation=left  Gain=0.128
  Gain12 : Gain  Orientation=left  Gain=1/0.01
  Gain15 : Gain  Gain=HSR
  Gain16 : Gain  Orientation=left  Gain=HTAUML
  Gain17 : Gain  Gain=HSL
  Gain18 : Gain  Gain=1/3
  Gain19 : Gain  Orientation=left  Gain=0.261
  Gain2 : Gain  Orientation=left  Gain=RAM
  Gain20 : Gain  Orientation=left  Gain=1/0.00355
  Gain21 : Gain  Gain=1/100
  Gain22 : Gain  Gain=FIS
  Gain23 : Gain  Gain=1/117
  Gain3 : Gain  Orientation=left  Gain=ANY
  Gain4 : Gain  Gain=1/CV
  Gain5 : Gain  Orientation=left  Gain=3.7
  Gain6 : Gain  Gain=0.574
  Gain7 : Gain  Gain=0.3986
  Gain8 : Gain  Gain=1/0.005
  Gain9 : Gain  Orientation=left  Gain=0.155
  Integrator : Integrator  InitialConditionSource=external
  Integrator1 : Integrator  InitialConditionSource=external
  Integrator2 : Integrator  Orientation=left  InitialConditionSource=external
  Integrator3 : Integrator  Orientation=left  InitialConditionSource=external
  Integrator4 : Integrator  InitialConditionSource=external
  MYOGRS Calculation : Subsystem
  Math Function : Math  Orientation=left  Operator=pow  SaturateOnIntegerOverflow=on
  Math Function2 : Math  Operator=pow  SaturateOnIntegerOverflow=on
  Math Function3 : Math  Operator=pow  SaturateOnIntegerOverflow=on
  PAMK Calculation : Subsystem
  Product : Product  Inputs=4  RndMeth=Zero
  Product1 : Product  Inputs=4  RndMeth=Zero
  Product10 : Product  RndMeth=Zero
  Product2 : Product  RndMeth=Zero
  Product3 : Product  Orientation=left  RndMeth=Zero
  Product4 : Product  Orientation=left  Inputs=4  RndMeth=Zero
  Product5 : Product  Orientation=left  RndMeth=Zero
  Product6 : Product  RndMeth=Zero
  Product7 : Product  Orientation=left  RndMeth=Zero
  Product8 : Product  Inputs=3  RndMeth=Zero
  Product9 : Product  Inputs=5  RndMeth=Zero
  QRN Calculation (FUN2) : Subsystem  Orientation=left
  RMULT1 Calculation : Subsystem  Orientation=left
  RPA Calculation : Subsystem  Orientation=left
  RPV Calculation : Subsystem
  RV1 Calculation : Subsystem  Orientation=left
  Saturation : Saturate  UpperLimit=inf  LowerLimit=0.0001
  Saturation1 : Saturate  UpperLimit=inf  LowerLimit=0.0001
  Saturation2 : Saturate  Orientation=up  UpperLimit=inf  LowerLimit=PR1LL
  Sum{,19,21,36} (4 alike) : Sum  Orientation=down
  Sum1 : Sum  Orientation=left  Inputs=-+|
  Sum10 : Sum  Orientation=down  Inputs=+-
  Sum{5,11,13..14,17,24,26,31} (8 alike) : Sum  Orientation=left  Inputs=|+-
  Sum12 : Sum  Orientation=left  Inputs=++|
  Sum15 : Sum  Orientation=left  Inputs=-+|
  Sum16 : Sum  Orientation=left  Inputs=++|
  Sum{4,6,9,18,30} (5 alike) : Sum  Inputs=|++
  Sum2 : Sum  Orientation=down  Inputs=+-----
  Sum20 : Sum  Orientation=down  Inputs=+-
  Sum22 : Sum  Orientation=up  Inputs=---++--
  Sum23 : Sum  Orientation=left  Inputs=|++
  Sum25 : Sum  Orientation=left  Inputs=|++
  Sum27 : Sum  Orientation=up  Inputs=+-
  Sum28 : Sum  Inputs=-+
  Sum3 : Sum  Inputs=|+-
  Sum32 : Sum  Inputs=|-+
  Sum33 : Sum  Inputs=|+-
  Sum34 : Sum  Inputs=+++
  Sum35 : Sum  Orientation=down  Inputs=++|
  Sum7 : Sum  Inputs=|+-
  Sum8 : Sum  Inputs=+-|
  Switch : Switch  Criteria=u2 > Threshold
  Switch2 : Switch  Criteria=u2 > Threshold
  Switch3 : Switch  Criteria=u2 > Threshold
  VVE : Outport
  PVS : Outport  Orientation=left  Port=2
  PRA : Outport  Port=3
  PLA : Outport  Port=4
  QLO : Outport  Port=5
  MYOGRS : Outport  Orientation=left  Port=6
  PA : Outport  Port=7
  QRO : Outport  Port=8
  PPA : Outport  Port=9
  RPV : Outport  Port=10
  RPA : Outport  Port=11
  QAO : Outport  Port=12
  BFN : Outport  Orientation=left  Port=13
  BFM : Outport  Port=14
  RVS : Outport  Orientation=left  Port=15
  PAMKRN : Outport  Port=16
  wires:
  VIM/1 -> Product/1, Product4/1, Gain5/1  "VIM"
  AUM/1 -> Product/2  "AUM"
  ANU/1 -> Product/3, Sum1/2  "ANU"
  ADHMV/1 -> Product/4  "ADHMV"
  Product/1 -> Product1/1
  Product1/1 -> CD47/1
  ATRRFB/1 -> CD47/2
  Math Function2/1 -> CD47/3, Math Function3/1  "PAM"
  CD47/1 -> Product2/2, Product3/1  "R1"
  ARM/1 -> Product2/1
  Product2/1 -> Gain/1
  Gain/1 -> Sum/1
  Gain1/1 -> Sum/2
  Product4/1 -> Gain1/1, RVS/1  "RVS"
  Sum/1 -> CD7/1  "RSN"
  AMM/1 -> Gain2/1
  Gain2/1 -> Product3/2
  PC/1 -> RV1 Calculation/1(PC), Sum36/2  "PC"
  RV1 Calculation/1(RV1) -> Product4/4  "RV1"
  AVE/1 -> Product4/2
  ANUVN/1 -> Product4/3
  Constant/1 -> Sum1/1
  Sum1/1 -> Gain3/1
  VVR/1 -> Sum2/2
  Gain3/1 -> Sum2/6
  VV7/1 -> Sum2/3
  VV6/1 -> Sum2/4
  ATRVFB/1 -> Sum2/5
  Sum2/1 -> Saturation/1  "VVE"
  Saturation/1 -> VVE/1, Sum3/1  "VVE"
  Constant1/1 -> Sum3/2
  Sum3/1 -> Gain4/1
  Gain4/1 -> Sum4/1
  Constant2/1 -> Sum4/2
  Sum4/1 -> Saturation1/1  "PVS"
  Saturation1/1 -> CD2/1, Sum5/1, Sum32/1, PVS/1  "PVS"
  Sum5/1 -> CD1/2  "PGV"
  Gain5/1 -> CD2/2  "3.7*VIM"
  CD2/1 -> Math Function/1
  Constant3/1 -> Math Function/2
  Saturation2/1 -> Sum5/2  "PR1"
  Math Function/1 -> CD3/2
  Constant4/1 -> CD3/1
  CD3/1 -> CD1/1  "RVG"
  Sum7/1 -> Integrator/1  "DVS"
  Constant5/1 -> Integrator/2
  Gain7/1 -> Sum6/2
  Sum8/1 -> Integrator1/1  "DRA"
  Constant6/1 -> Integrator1/2
  Constant7/1 -> Sum10/2
  Sum10/1 -> Gain8/1  "VRE"
  Gain8/1 -> Saturation2/1, QRN Calculation (FUN2)/1(PRA), PRA/1, Sum33/2  "PRA"
  QRN Calculation (FUN2)/1(QRN) -> Product5/2  "QRN"
  AU/1 -> QRN Calculation (FUN2)/2(AU), Sum24/1  "AU"
  Product5/1 -> Sum11/1, QRO/1, Sum8/2, Damping1/1(QRO)  "QRO"
  Sum11/1 -> Integrator2/1  "DPA"
  Constant8/1 -> Integrator2/2
  Gain9/1 -> Sum12/1
  Constant9/1 -> Sum13/2
  Sum13/1 -> Gain10/1  "VPE"
  Gain10/1 -> Sum14/1, CD68/1, RPA Calculation/1(PPA), PPA/1  "PPA"
  Sum14/1 -> CD4/2  "PGL"
  CD4/1 -> Damping/2(QPO_a)  "QPO"
  Gain11/1 -> Sum16/1
  Sum17/1 -> Gain12/1  "VLE"
  Constant10/1 -> Sum17/2
  Sum15/1 -> Integrator3/1  "DLA"
  Constant11/1 -> Integrator3/2
  Gain12/1 -> PLA/1, Sum23/1, RPV Calculation/1(PLA), Sum14/2, Sum28/2  "PLA"
  RPV Calculation/1(RPV) -> RPV/1, Sum19/1  "RPV"
  Sum19/1 -> CD4/1  "RPT"
  OSA/1 -> Product6/1  "OSA"
  AUH/1 -> Product8/1, Product9/5, Product6/2  "AUH"
  Product6/1 -> CD68/2, CD8/2  "AUH*OSA"
  CD68/1 -> FUN3/1(PP2)  "PP2"
  FUN3/1(RVM) -> CD72/2  "RVM"
  HMD/1 -> Product8/2, Product9/4  "HMD"
  HPR/1 -> Product8/3
  Product8/1 -> CD72/3  "AUH*HMD*HPR"
  Constant16/1 -> Sum20/2, CD70/2  "QRF"
  Constant17/1 -> Sum20/1
  Sum20/1 -> CD72/1
  Sum22/1 -> Gain19/1, Gain11/1, Gain6/1, Gain9/1, Gain7/1  "VBD"
  CD72/1 -> Gain15/1
  Gain15/1 -> Sum21/2
  Sum21/1 -> Product5/1  "HPEF"
  CD70/1 -> CD71/2
  CD71/1 -> Sum21/1  "QRF*QLO/QLN"
  VP/1 -> Sum22/4
  VRC/1 -> Sum22/5
  Constant18/1 -> Sum23/2
  Constant19/1 -> Sum24/2, Sum25/2
  Sum24/1 -> Gain16/1
  Gain16/1 -> Sum25/1
  Sum23/1 -> Product7/1
  Sum25/1 -> Product7/2
  Product7/1 -> Sum26/1
  Constant20/1 -> Sum26/2
  Sum26/1 -> FUN4/1(PLA1)  "PLA1"
  FUN4/1(QLN) -> Product9/3, CD71/1  "QLN"
  HPL/1 -> Product9/2
  FUN1/1(LVM) -> Product9/1  "LVM"
  Product9/1 -> Gain17/1
  Gain17/1 -> Switch/3, Sum18/2  "QLO"
  Sum27/1 -> Integrator4/1  "DAS"
  Sum28/1 -> Gain18/1
  Gain18/1 -> Switch/2, Sum18/1  "QLO1"
  Switch/1 -> Sum27/1, CD70/1, Sum15/1, Damping/1(QLO), QLO/1  "QLO"
  Gain19/1 -> Sum30/2
  Constant22/1 -> Sum31/2
  Sum31/1 -> Gain20/1  "VAE"
  Gain20/1 -> Sum28/1, Sum32/2, Gain21/1, PA/1, Sum36/1, Sum33/1, CD8/1  "PA"
  Gain21/1 -> Math Function2/1, PAMK Calculation/1(PA/100)  "PA/100"
  Sum32/1 -> CD6/1, CD7/2  "PGS"
  Product3/1 -> CD6/2  "RSM"
  CD7/1 -> Sum34/2, BFN/1, RMULT1 Calculation/1(BFN)  "BFN"
  CD6/1 -> Sum34/3, BFM/1, RMULT1 Calculation/2(BFM)  "BFM"
  Sum33/1 -> Gain22/1
  RBF/1 -> Sum34/1
  Sum34/1 -> Sum35/2  "SYSFLO"
  Gain22/1 -> Sum35/1  "FISFLO"
  Sum35/1 -> Sum7/1, Sum27/2, QAO/1  "QAO"
  CD8/1 -> FUN1/1(PA2)  "PA2"
  Sum36/1 -> Gain23/1
  Constant25/1 -> Math Function3/2
  Gain23/1 -> Product10/1
  Math Function3/1 -> Product10/2
  Constant31/1 -> Switch2/2
  Constant32/1 -> Switch2/3
  Constant35/1 -> Switch3/2
  Switch2/1 -> Product1/4, Switch3/1  "PAMK"
  PAMK Calculation/1(PAMK) -> Switch2/1
  Switch3/1 -> PAMKRN/1  "PAMKRN"
  Constant33/1 -> Switch3/3
  Constant23/1 -> Math Function2/2
  RMULT1 Calculation/1(RMULT1) -> Product1/2  "RMULT1"
  RPA Calculation/1(RPA) -> RPA/1, Sum19/2  "RPA"
  Constant21/1 -> Integrator4/2
  Product10/1 -> MYOGRS Calculation/1(TENS1)  "TENS1"
  MYOGRS Calculation/1(MYOGRS) -> Product1/3, MYOGRS/1  "MYOGRS"
  CD1/1 -> Damping1/2(QVO_a)  "QVO"
  Integrator/1 -> Sum6/1
  Sum6/1 -> Sum2/1, Sum22/7  "VVS"
  Gain6/1 -> Sum9/2
  Integrator1/1 -> Sum9/1
  Sum9/1 -> Sum10/1, Sum22/6  "VRA"
  Integrator3/1 -> Sum16/2
  Sum16/1 -> Sum17/1, Sum22/2  "VLA"
  Integrator4/1 -> Sum30/1
  Sum30/1 -> Sum31/1, Sum22/1  "VAS"
  Integrator2/1 -> Sum12/2
  Sum12/1 -> Sum13/1, Sum22/3  "VPA"
  Sum18/1 -> Switch/1
  Damping1/1(QVO) -> Sum8/1, Sum7/2  "QVO"
  Damping/1(QPO) -> Sum15/2, Sum11/2  "QPO"

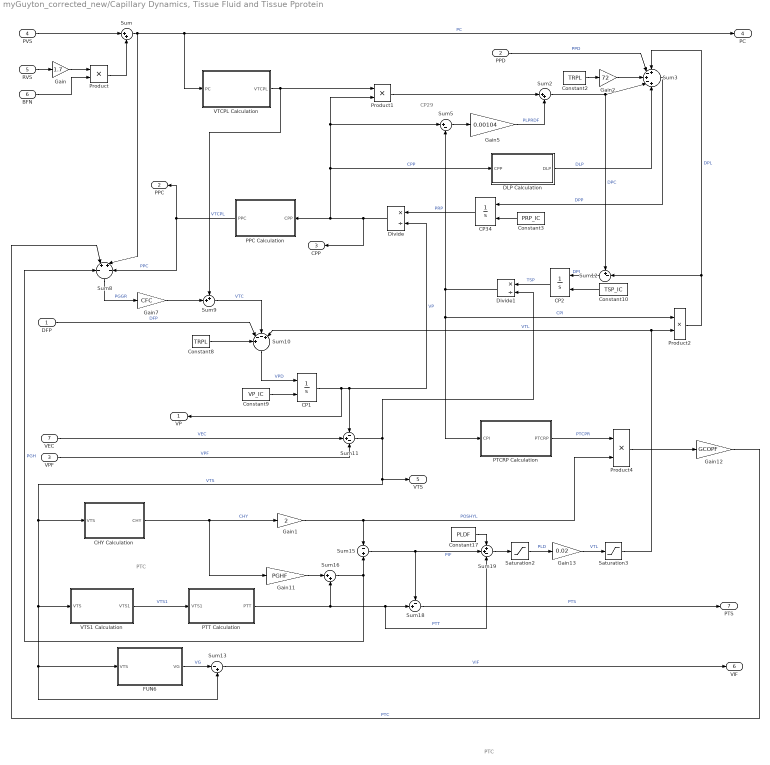
== system myGuyton_corrected_new/Capillary Dynamics, Tissue Fluid and Tissue Pprotein  ==
  note: CP29
  note: PTC
  note: PTC
  DFP : Inport
  PPD : Inport  Port=2
  VPF : Inport  Port=3
  PVS : Inport  Port=4
  RVS : Inport  Port=5
  BFN : Inport  Port=6
  VEC : Inport  Port=7
  CHY Calculation : Subsystem
  CP1 : Integrator  InitialConditionSource=external
  CP2 : Integrator  Orientation=left  InitialConditionSource=external
  CP34 : Integrator  Orientation=left  InitialConditionSource=external
  Constant10 : Constant  Orientation=left  Value=TSP_IC
  Constant17 : Constant  Value=PLDF
  Constant2 : Constant  Value=TRPL
  Constant3 : Constant  Orientation=left  Value=PRP_IC
  Constant8 : Constant  Value=TRPL
  Constant9 : Constant  Value=VP_IC
  DLP Calculation : Subsystem
  Divide : Product  Orientation=left  Inputs=*/  OutScaling=2^-10
  Divide1 : Product  Orientation=left  Inputs=*/  OutScaling=2^-10
  FUN6 : Subsystem
      mask Display: plot([0 12 15 18 21 24],[0 11.4 14 16 17.3 18])
  Gain : Gain  Gain=1.7
  Gain1 : Gain  Gain=2
  Gain11 : Gain  Gain=PGHF
  Gain12 : Gain  Gain=GCOPF
  Gain13 : Gain  Gain=0.02
  Gain2 : Gain  Gain=72
  Gain5 : Gain  Gain=0.00104
  Gain7 : Gain  Gain=CFC
  PPC Calculation : Subsystem  Orientation=left
  PTCRP Calculation : Subsystem
  PTT Calculation : Subsystem
  Product{,1..2,4} (4 alike) : Product  RndMeth=Zero
  Saturation2 : Saturate  UpperLimit=7  LowerLimit=-inf
  Saturation3 : Saturate  UpperLimit=inf  LowerLimit=0
  Sum : Sum  Inputs=|++
  Sum10 : Sum  Orientation=down  Inputs=+--+|
  Sum11 : Sum  Inputs=-+-
  Sum12 : Sum  Orientation=left  Inputs=+-|
  Sum13 : Sum  Inputs=|-+
  Sum15 : Sum  Inputs=-+
  Sum16 : Sum  Inputs=|++
  Sum18 : Sum  Inputs=-+|
  Sum19 : Sum  Inputs=++-
  Sum2 : Sum  Inputs=|++
  Sum3 : Sum  Inputs=+-+-+
  Sum5 : Sum  Inputs=|+-
  Sum8 : Sum  Orientation=down  Inputs=-++-
  Sum9 : Sum  Inputs=++|
  VTCPL Calculation : Subsystem
  VTS1 Calculation : Subsystem
  VP : Outport  Orientation=left
  PPC : Outport  Orientation=left  Port=2
  CPP : Outport  Orientation=left  Port=3
  PC : Outport  Port=4
  VTS : Outport  Port=5
  VIF : Outport  Port=6
  PTS : Outport  Port=7
  wires:
  RVS/1 -> Gain/1
  Gain/1 -> Product/1
  BFN/1 -> Product/2
  PVS/1 -> Sum/1
  Product/1 -> Sum/2
  Sum/1 -> PC/1, VTCPL Calculation/1(PC), Sum8/3  "PC"
  VTCPL Calculation/1(VTCPL) -> Product1/1, Sum9/1  "VTCPL"
  Product1/1 -> Sum2/1
  Gain5/1 -> Sum2/2  "PLPRDF"
  Product2/1 -> Sum3/1, Sum12/2  "DPL"
  Sum3/1 -> CP34/1  "DPP"
  Constant2/1 -> Gain2/1
  Constant3/1 -> CP34/2
  CP34/1 -> Divide/1  "PRP"
  Divide/1 -> PPC Calculation/1(CPP), Sum5/1, Product1/2, DLP Calculation/1(CPP), CPP/1  "CPP"
  PPC Calculation/1(PPC) -> Sum8/4, PPC/1  "PPC"
  Sum5/1 -> Gain5/1
  Gain2/1 -> Sum3/3
  PPD/1 -> Sum3/2  "PPD"
  DLP Calculation/1(DLP) -> Sum3/5  "DLP"
  Sum8/1 -> Gain7/1  "PGGR"
  Gain7/1 -> Sum9/2
  Sum9/1 -> Sum10/3  "VTC"
  DFP/1 -> Sum10/2  "DFP"
  Constant8/1 -> Sum10/1
  Sum10/1 -> CP1/1  "VPD"
  CP1/1 -> Sum11/1, Divide/2, VP/1  "VP"
  Constant9/1 -> CP1/2
  VEC/1 -> Sum11/2  "VEC"
  VPF/1 -> Sum11/3  "VPF"
  Sum11/1 -> VTS1 Calculation/1(VTS), Sum13/2, FUN6/1(VTS), CHY Calculation/1(VTS), VTS/1, Divide1/2  "VTS"
  Sum12/1 -> CP2/1  "DPI"
  Constant10/1 -> CP2/2
  CP2/1 -> Divide1/1  "TSP"
  Divide1/1 -> Sum5/2, Product2/1, PTCRP Calculation/1(CPI)  "CPI"
  FUN6/1(VG) -> Sum13/1  "VG"
  Sum13/1 -> VIF/1  "VIF"
  CHY Calculation/1(CHY) -> Gain11/1, Gain1/1  "CHY"
  PTCRP Calculation/1(PTCRP) -> Product4/1  "PTCPR"
  Gain1/1 -> Sum15/1, Product4/2  "POSHYL"
  Gain11/1 -> Sum16/1
  PTT Calculation/1(PTT) -> Sum16/2, Sum18/2, Sum19/3  "PTT"
  Sum16/1 -> Sum15/2, Sum8/1  "PGH"
  Sum15/1 -> Sum18/1, Sum19/2  "PIF"
  Product4/1 -> Gain12/1
  Gain12/1 -> Sum8/2  "PTC"
  VTS1 Calculation/1(VTS1) -> PTT Calculation/1(VTS1)  "VTS1"
  Sum18/1 -> PTS/1  "PTS"
  Sum19/1 -> Saturation2/1
  Saturation2/1 -> Gain13/1  "PLD"
  Gain13/1 -> Saturation3/1  "VTL"
  Saturation3/1 -> Product2/2, Sum10/4  "VTL"
  Constant17/1 -> Sum19/1
  Sum2/1 -> Sum12/1, Sum3/4  "DPC"

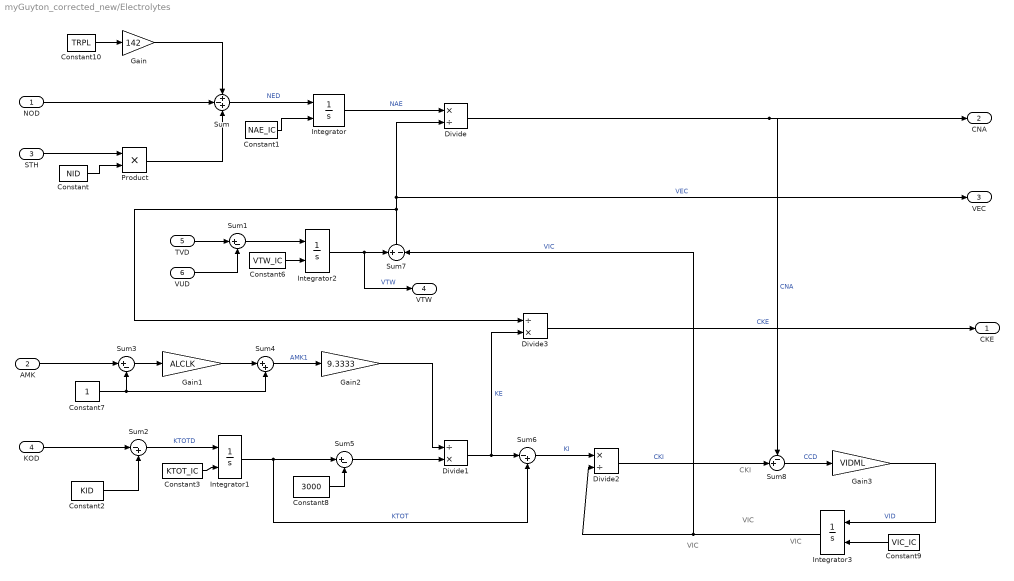
== system myGuyton_corrected_new/Electrolytes ==
  note: CKI
  note: VIC
  note: VIC
  note: VIC
  NOD : Inport
  AMK : Inport  Port=2
  STH : Inport  Port=3
  KOD : Inport  Port=4
  TVD : Inport  Port=5
  VUD : Inport  Port=6
  Constant : Constant  Value=NID
  Constant1 : Constant  Value=NAE_IC
  Constant10 : Constant  Value=TRPL
  Constant2 : Constant  Value=KID
  Constant3 : Constant  Value=KTOT_IC
  Constant6 : Constant  Value=VTW_IC
  Constant7 : Constant
  Constant8 : Constant  Value=3000
  Constant9 : Constant  Orientation=left  Value=VIC_IC
  Divide : Product  Inputs=*/  OutScaling=2^-10
  Divide1 : Product  Inputs=/*  OutScaling=2^-10
  Divide2 : Product  Inputs=*/  OutScaling=2^-10
  Divide3 : Product  Inputs=/*  OutScaling=2^-10
  Gain : Gain  Gain=142
  Gain1 : Gain  Gain=ALCLK
  Gain2 : Gain  Gain=9.3333
  Gain3 : Gain  Gain=VIDML
  Integrator : Integrator  InitialConditionSource=external
  Integrator1 : Integrator  InitialConditionSource=external
  Integrator2 : Integrator  InitialConditionSource=external
  Integrator3 : Integrator  Orientation=left  InitialConditionSource=external
  Product : Product  RndMeth=Zero
  Sum : Sum  Inputs=+-+
  Sum1 : Sum  Inputs=|+-
  Sum2 : Sum  Inputs=|-+
  Sum3 : Sum  Inputs=|+-
  Sum4 : Sum  Inputs=|++
  Sum5 : Sum  Inputs=|+-
  Sum6 : Sum  Inputs=|-+
  Sum7 : Sum  Orientation=up  Inputs=+-
  Sum8 : Sum  Inputs=-+|
  CKE : Outport
  CNA : Outport  Port=2
  VEC : Outport  Port=3
  VTW : Outport  Port=4
  wires:
  Constant10/1 -> Gain/1
  STH/1 -> Product/1
  Constant/1 -> Product/2
  Gain/1 -> Sum/1
  NOD/1 -> Sum/2
  Product/1 -> Sum/3
  Sum/1 -> Integrator/1  "NED"
  Constant1/1 -> Integrator/2
  Integrator/1 -> Divide/1  "NAE"
  Divide/1 -> CNA/1, Sum8/1  "CNA"
  KOD/1 -> Sum2/1
  Constant2/1 -> Sum2/2
  Sum2/1 -> Integrator1/1  "KTOTD"
  Constant3/1 -> Integrator1/2
  Integrator1/1 -> Sum5/1, Sum6/2  "KTOT"
  Constant8/1 -> Sum5/2
  Sum5/1 -> Divide1/2
  Sum6/1 -> Divide2/1  "KI"
  TVD/1 -> Sum1/1
  VUD/1 -> Sum1/2
  Sum1/1 -> Integrator2/1
  Constant6/1 -> Integrator2/2
  Integrator2/1 -> Sum7/1, VTW/1  "VTW"
  Sum7/1 -> Divide3/1, Divide/2, VEC/1  "VEC"
  Divide2/1 -> Sum8/2  "CKI"
  Sum8/1 -> Gain3/1  "CCD"
  Gain3/1 -> Integrator3/1  "VID"
  Constant9/1 -> Integrator3/2
  Integrator3/1 -> Sum7/2, Divide2/2  "VIC"
  AMK/1 -> Sum3/1
  Constant7/1 -> Sum3/2, Sum4/2
  Sum3/1 -> Gain1/1
  Gain1/1 -> Sum4/1
  Sum4/1 -> Gain2/1  "AMK1"
  Gain2/1 -> Divide1/1
  Divide1/1 -> Sum6/1, Divide3/2  "KE"
  Divide3/1 -> CKE/1  "CKE"

== system myGuyton_corrected_new/Heart Hypertrophy or Deteoration ==
  PA : Inport
  QAO : Inport  Port=2
  PPA : Inport  Port=3
  POT : Inport  Port=4
  Constant1 : Constant  Value=10
  Constant4 : Constant  Value=Z13
  Constant7 : Constant  Value=Z13
  Constant8 : Constant  Value=HMD_IC
  Gain1 : Gain  Gain=1/500
  Gain2 : Gain  Gain=1/HSL
  Gain3 : Gain  Gain=1/75
  Gain4 : Gain  Gain=DHDTR
  Gain5 : Gain  Gain=1/HSR
  HH13 : Integrator  InitialConditionSource=external
  HH14 : Saturate  UpperLimit=1  LowerLimit=-inf  LinearizeAsGain=off
  HH1A : Product  RndMeth=Zero
  HH2 : Math  Operator=pow  SaturateOnIntegerOverflow=on
  HH6A : Product  RndMeth=Zero
  HH7 : Math  Operator=pow  SaturateOnIntegerOverflow=on
  Hypertr. Eff. on LV : Subsystem
      mask Display: dpoly([0 1],[57600 1],'s')
  Hypertr. Eff. on RV : Subsystem
      mask Display: dpoly([0 1],[57600 1],'s')
  Sum : Sum  Inputs=|+-
  HPL : Outport
  HPR : Outport  Port=2
  HMD : Outport  Port=3
  wires:
  QAO/1 -> HH1A/2, HH6A/1
  HH7/1 -> Hypertr. Eff. on RV/1(In1)
  Constant7/1 -> HH7/2
  Gain5/1 -> HH7/1
  Gain3/1 -> Gain5/1
  HH6A/1 -> Gain3/1
  HH2/1 -> Hypertr. Eff. on LV/1(In1)
  Constant4/1 -> HH2/2
  Gain2/1 -> HH2/1
  Gain1/1 -> Gain2/1
  HH1A/1 -> Gain1/1
  HH13/1 -> HH14/1  "HMD"
  Gain4/1 -> HH13/1  "DHM"
  Sum/1 -> Gain4/1
  Constant1/1 -> Sum/2
  POT/1 -> Sum/1
  PA/1 -> HH1A/1
  Hypertr. Eff. on LV/1(HPL) -> HPL/1
  Hypertr. Eff. on RV/1(HPR) -> HPR/1
  PPA/1 -> HH6A/2
  HH14/1 -> HMD/1
  Constant8/1 -> HH13/2

== system myGuyton_corrected_new/Heart Rate and Stroke Volume ==
  QLO : Inport
  AUR : Inport  Port=2
  HMD : Inport  Port=3
  Constant : Constant  Value=0.5
  Constant1 : Constant
  Constant2 : Constant
  Constant3 : Constant  Value=PR1LL
  Divide : Product  Inputs=*/  OutScaling=2^-10
  Gain : Gain  Gain=5
  Gain1 : Gain  Gain=72
  HR5 : Gain  Gain=0.5
  HR7 : Product  RndMeth=Zero
  Math Function : Math  Operator=pow  SaturateOnIntegerOverflow=on
  Sum : Sum  Inputs=|+-
  Sum1 : Sum  Inputs=|++
  Sum2 : Sum  Inputs=|++
  SVO : Outport
  HR : Outport  Port=2
  wires:
  Constant/1 -> Math Function/2
  Math Function/1 -> Gain/1
  Constant1/1 -> Sum/2
  Sum/1 -> HR5/1
  Constant2/1 -> Sum1/2
  HR5/1 -> Sum1/1
  Gain1/1 -> Sum2/1
  Gain/1 -> Sum2/2
  Sum2/1 -> HR7/1
  Sum1/1 -> HR7/2
  HR7/1 -> Divide/2, HR/1  "HR"
  HMD/1 -> Sum/1
  QLO/1 -> Divide/1
  Divide/1 -> SVO/1
  AUR/1 -> Gain1/1
  Constant3/1 -> Math Function/1
